simulink model "PCA_6m"  (R2018b)
settings: Solver=VariableStepAuto  StartTime=0.0  StopTime=20  RelTol=1e-8
values from neighbouring files (symbols this model uses):
  G = [G1 G2 0 0]    [PCA_6.m]    (also in PCA_6b.m; PCA_6d.m = 1.0e+03 *[-6.4032   -2.2650   -1.0265   -0.2756]; TH3_7.m = [27 271 915]; TH3_7b.m = place(A, B, poles))
  G0 = Bnum*E    [PCA_6d.m]    (also in TH3_7b.m; TH3_8b.m)
settings Model: Creator=friedlan  LastModifiedBy=ohara
settings DebuggingCC: LibraryContextMissingDiagnostic=none
settings SFSimCC: SimUseLocalCustomCode=off
settings RTWCC: RTWUseLocalCustomCode=off

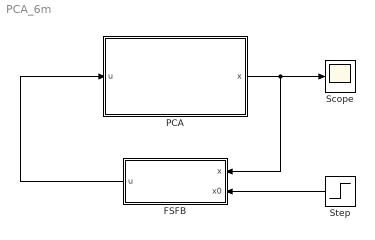
== system PCA_6m ==
  FSFB : Subsystem
  PCA : Subsystem
  Scope : Scope
  Step : Step  SampleTime=0
  wires:
  PCA/1(x) -> FSFB/1(x), Scope/1
  FSFB/1(u) -> PCA/1(u)
  Step/1 -> FSFB/2(x0)

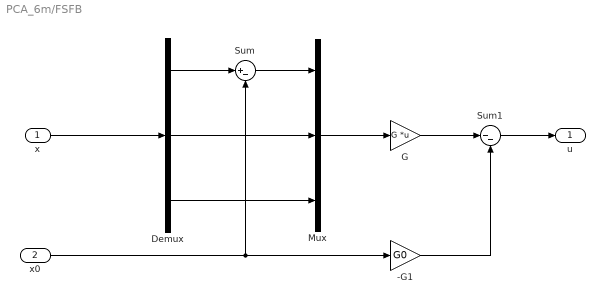
== system PCA_6m/FSFB ==
  x : Inport
  x0 : Inport  Port=2
  -G1 : Gain  Gain=G0
  Demux : Demux  Outputs=3
  G : Gain  Gain=G  Multiplication=Matrix(K*u)
  Mux : Mux  Inputs=3
  Sum : Sum  Inputs=|+-
  Sum1 : Sum  Inputs=|--
  u : Outport
  wires:
  x/1 -> Demux/1
  Mux/1 -> G/1
  Demux/1 -> Sum/1
  x0/1 -> -G1/1, Sum/2
  Sum/1 -> Mux/1
  G/1 -> Sum1/1
  -G1/1 -> Sum1/2
  Sum1/1 -> u/1
  Demux/2 -> Mux/2
  Demux/3 -> Mux/3

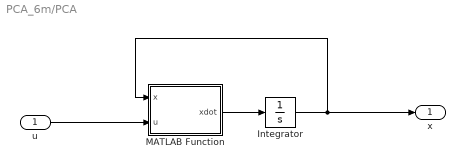
== system PCA_6m/PCA ==
  u : Inport
  Integrator : Integrator  InitialCondition=[0;0;0;0]
  MATLAB Function : MATLAB Function  TreatAsAtomicUnit=on
  x : Outport
  wires:
  u/1 -> MATLAB Function/2(u)
  MATLAB Function/1(xdot) -> Integrator/1
  Integrator/1 -> x/1, MATLAB Function/1(x)

== matlab function PCA_6m/PCA/MATLAB Function ==
  data: x input; u input; xdot output
function xdot  = PCA(x, u)
a = 4;
b = 1;
M = 1;
m = 0.4;
g = 9.81;
L = 0.25*M;
xdot1 = x(3);
xdot2 = x(4);
xdot3 = -a*x(3) - ((m*g)/M)*x(2) + b*u;
xdot4 = (a/L)*x(3) - (M+m)*(g/(M*L))*x(2) - (b/L)*u;
xdot  = [xdot1; xdot2; xdot3; xdot4];
